simulink subsystem "thermal_controller_standalone"  (R2022b)
settings: Solver=VariableStepAuto  StartTime=0.0  StopTime=10.0  RelTol=1e-3
libraries: slpidlib x1
settings Model: Creator=michael.roesch  LastModifiedBy=stefan.notter

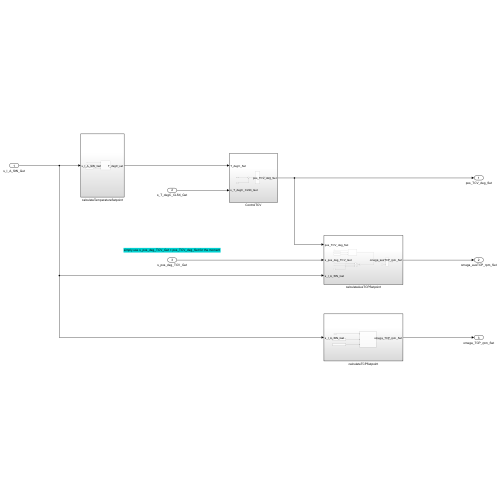
[thumbnail: Simulink's stored preview of the top-level diagram]
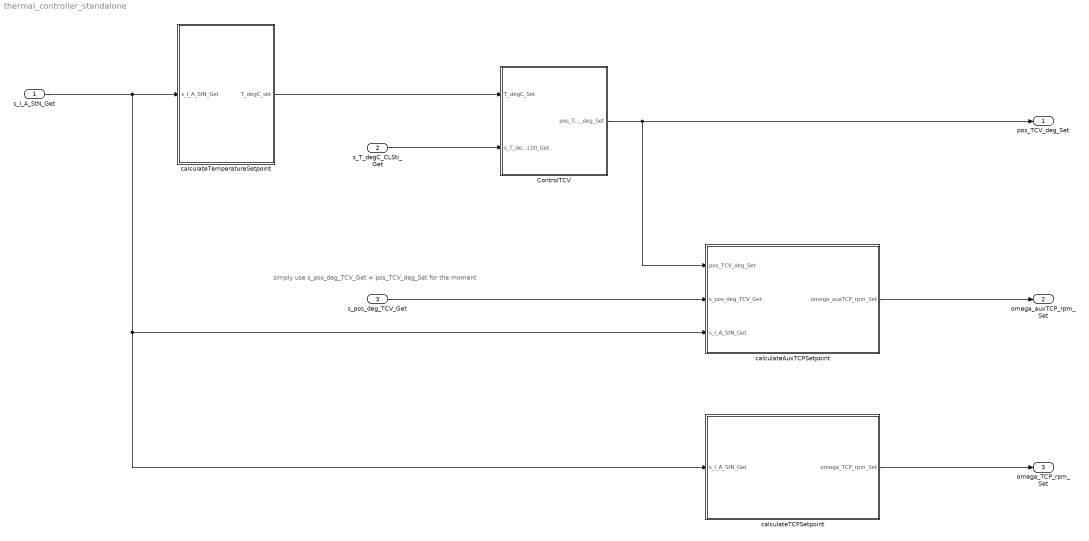
== system thermal_controller_standalone ==
  note: simply use s_pos_deg_TCV_Get = pos_TCV_deg_Set for the moment
  s_I_A_StN_Get : Inport
  s_T_degC_CLSti_Get : Inport  Port=2
  s_pos_deg_TCV_Get : Inport  Port=3
  ControlTCV : Subsystem
  calculateAuxTCPSetpoint : Subsystem
  calculateTCPSetpoint : Subsystem
  calculateTemperatureSetpoint : Subsystem
  pos_TCV_deg_Set : Outport
  omega_auxTCP_rpm_Set : Outport  Port=2
  omega_TCP_rpm_Set : Outport  Port=3
  wires:
  calculateTemperatureSetpoint/1(T_degC_set) -> ControlTCV/1(T_degC_Set)
  calculateTCPSetpoint/1(omega_TCP_rpm_Set) -> omega_TCP_rpm_Set/1
  calculateAuxTCPSetpoint/1(omega_auxTCP_rpm_Set) -> omega_auxTCP_rpm_Set/1
  ControlTCV/1(pos_TCV_deg_Set) -> pos_TCV_deg_Set/1, calculateAuxTCPSetpoint/1(pos_TCV_deg_Set)
  s_I_A_StN_Get/1 -> calculateTCPSetpoint/1(s_I_A_StN_Get), calculateAuxTCPSetpoint/3(s_I_A_StN_Get), calculateTemperatureSetpoint/1(s_I_A_StN_Get)
  s_T_degC_CLSti_Get/1 -> ControlTCV/2(s_T_degC_CLSti_Get)
  s_pos_deg_TCV_Get/1 -> calculateAuxTCPSetpoint/2(s_pos_deg_TCV_Get)

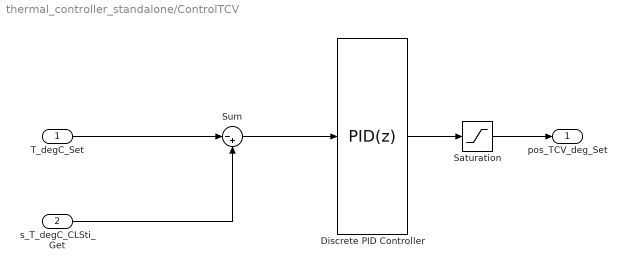
== system thermal_controller_standalone/ControlTCV ==
  T_degC_Set : Inport
  s_T_degC_CLSti_Get : Inport  Port=2
  Discrete PID Controller : slpidlib/PID Controller  Controller=PID  Form=Parallel  TimeDomain=Discrete-time  UseExternalTs=off  SampleTime=-1  IntegratorMethod=Forward Euler  FilterMethod=Forward Euler  ControllerParametersSource=internal  P=500  I=1  UseKiTs=on  D=0  N=0  UseFilter=on  TunerSelectOption=Transfer Function Based (PID Tuner App)  InitialConditionSource=internal  InitialConditionForIntegrator=0  InitialConditionForFilter=0  DifferentiatorICPrevScaledInput=0  ExternalReset=none  TrackingMode=off  Kt=1  LimitOutput=off  SatLimitsSource=internal  UpperSaturationLimit=90  LowerSaturationLimit=25  LinearizeAsGain=on  AntiWindupMode=clamping  Kb=1  LimitIntegrator=off  UpperIntegratorSaturationLimit=inf  LowerIntegratorSaturationLimit=-inf  POutMin=[]  POutMax=[]  IOutMin=[]  IOutMax=[]  DOutMin=[]  DOutMax=[]  NOutMin=[]  NOutMax=[]  SumOutMin=[]  SumOutMax=[]  SaturationOutMin=[]  SaturationOutMax=[]  PParamMin=[]  PParamMax=[]  IParamMin=[]  IParamMax=[]  DParamMin=[]  DParamMax=[]  NParamMin=[]  NParamMax=[]  KbParamMin=[]  KbParamMax=[]  KtParamMin=[]  KtParamMax=[]  KbOutMin=[]  KbOutMax=[]  KtOutMin=[]  KtOutMax=[]  IntegratorOutMin=[]  IntegratorOutMax=[]  FilterOutMin=[]  FilterOutMax=[]  SumI1OutMin=[]  SumI1OutMax=[]  SumI2OutMin=[]  SumI2OutMax=[]  SumI3OutMin=[]  SumI3OutMax=[]  SumI4OutMin=[]  SumI4OutMax=[]  SumDOutMin=[]  SumDOutMax=[]  DifferentiatorOutMin=[]  DifferentiatorOutMax=[]  FilterDiffOutCoefMin=[]  FilterDiffOutCoefMax=[]  ReciprocalOutMin=[]  ReciprocalOutMax=[]  SumDenOutMin=[]  SumDenOutMax=[]  SumNumOutMin=[]  SumNumOutMax=[]  DivideOutMin=[]  DivideOutMax=[]  UdiffTsProdOutMin=[]  UdiffTsProdOutMax=[]  NTsProdOutMin=[]  NTsProdOutMax=[]  UintegralTsProdOutMin=[]  UintegralTsProdOutMax=[]  UngainTsProdOutMin=[]  UngainTsProdOutMax=[]  ClampingZeroOutDataTypeStr=Inherit: Inherit via back propagation  ClampingZeroOutMin=[]  ClampingZeroOutMax=[]  FilterDenConstantOutDataTypeStr=Inherit: Inherit via back propagation  FilterDenConstantOutMin=[]  FilterDenConstantOutMax=[]  PCopyOutDataTypeStr=Inherit: Inherit via back propagation  PCopyOutMin=[]  PCopyOutMax=[]  NCopyOutDataTypeStr=Inherit: Inherit via back propagation  NCopyOutMin=[]  NCopyOutMax=[]  IntegratorContinuousStateAttributes=''  IntegratorStateMustResolveToSignalObject=off  IntegratorRTWStateStorageClass=Auto  FilterContinuousStateAttributes=''  FilterStateMustResolveToSignalObject=off  FilterRTWStateStorageClass=Auto  ParallelPVariant=InternalParameters  IdealPVariant=Disabled  IVariant=InternalParameters  DVariant=InternalParameters  IntegratorVariant=Discrete  SatVariant=Disabled  AWVariant=Passthrough  PCopyVariant=Disabled  TRVariant=Disabled  FdbkBlocksVariant=Forward  IdealPFdbkVariant=Disabled  SatFdbkVariant=Disabled  DerivativeFilterVariant=ForwardEulerFilter  NVariant=InternalParameters  NCopyVariant=Disabled  FilterICVariant=InternalICsFilter  IntegratorICVariant=InternalICs  ExternalResetVariant=Disabled  TRSumVariant=Passthrough  SumFdbkVariant=Disabled  SumVariant=Sum_PID  TsampFilterVariant=InternalTs  TsampNgainVariant=Passthrough  TsampIntegralVariant=Passthrough  ExternalSaturationOutDataTypeStr=Inherit: Same as second input
      settings: LibrarySourceBlock=simulink/Discrete/Discrete PID Controller
  Saturation : Saturate  UpperLimit=90  LowerLimit=25
  Sum : Sum  Inputs=|-+
  pos_TCV_deg_Set : Outport
  wires:
  T_degC_Set/1 -> Sum/1
  Discrete PID Controller/1 -> Saturation/1
  Sum/1 -> Discrete PID Controller/1
  s_T_degC_CLSti_Get/1 -> Sum/2
  Saturation/1 -> pos_TCV_deg_Set/1

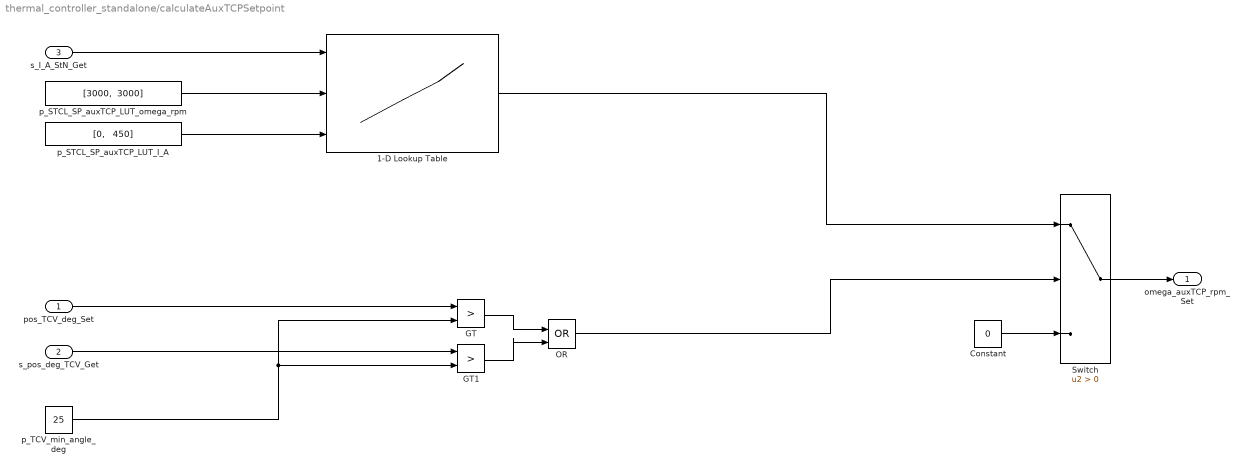
== system thermal_controller_standalone/calculateAuxTCPSetpoint ==
  pos_TCV_deg_Set : Inport
  s_pos_deg_TCV_Get : Inport  Port=2
  s_I_A_StN_Get : Inport  Port=3
  1-D Lookup Table : Lookup_n-D  NumberOfTableDimensions=1  BreakpointsForDimension1Source=Input port  BreakpointsForDimension1=[-5:5]  TableSource=Input port  Table=tanh([-5:5])  InternalRulePriority=Speed  RndMeth=Simplest
      settings: InputPortMap=u0,p221,p5
  Constant : Constant  Value=0
  GT : RelationalOperator  Operator=>  OutDataTypeStr=boolean  RndMeth=Simplest  InputSameDT=off
  GT1 : RelationalOperator  Operator=>  OutDataTypeStr=boolean  RndMeth=Simplest  InputSameDT=off
  OR : Logic  Operator=OR  IconShape=distinctive  AllPortsSameDT=off  OutDataTypeStr=boolean
  Switch : Switch  Criteria=u2 > Threshold  SaturateOnIntegerOverflow=off  InputSameDT=off
  p_STCL_SP_auxTCP_LUT_I_A : Constant  Value="[0,   450]"
  p_STCL_SP_auxTCP_LUT_omega_rpm : Constant  Value="[3000,  3000]"
  p_TCV_min_angle_deg : Constant  Value=25
  omega_auxTCP_rpm_Set : Outport
  wires:
  Constant/1 -> Switch/3
  OR/1 -> Switch/2
  GT1/1 -> OR/2
  GT/1 -> OR/1
  pos_TCV_deg_Set/1 -> GT/1
  s_I_A_StN_Get/1 -> 1-D Lookup Table/1
  Switch/1 -> omega_auxTCP_rpm_Set/1
  1-D Lookup Table/1 -> Switch/1
  p_STCL_SP_auxTCP_LUT_omega_rpm/1 -> 1-D Lookup Table/2
  p_STCL_SP_auxTCP_LUT_I_A/1 -> 1-D Lookup Table/3
  s_pos_deg_TCV_Get/1 -> GT1/1
  p_TCV_min_angle_deg/1 -> GT/2, GT1/2

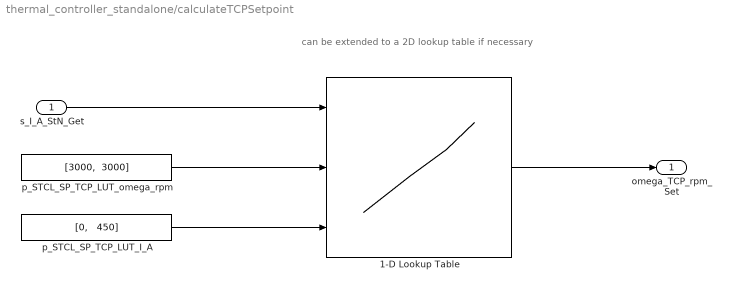
== system thermal_controller_standalone/calculateTCPSetpoint ==
  note: can be extended to a 2D lookup table if necessary
  s_I_A_StN_Get : Inport
  1-D Lookup Table : Lookup_n-D  NumberOfTableDimensions=1  BreakpointsForDimension1Source=Input port  BreakpointsForDimension1=[-5:5]  TableSource=Input port  Table=tanh([-5:5])  InternalRulePriority=Speed  RndMeth=Simplest
      settings: InputPortMap=u0,p221,p5
  p_STCL_SP_TCP_LUT_I_A : Constant  Value="[0,   450]"
  p_STCL_SP_TCP_LUT_omega_rpm : Constant  Value="[3000,  3000]"
  omega_TCP_rpm_Set : Outport
  wires:
  1-D Lookup Table/1 -> omega_TCP_rpm_Set/1
  s_I_A_StN_Get/1 -> 1-D Lookup Table/1
  p_STCL_SP_TCP_LUT_omega_rpm/1 -> 1-D Lookup Table/2
  p_STCL_SP_TCP_LUT_I_A/1 -> 1-D Lookup Table/3

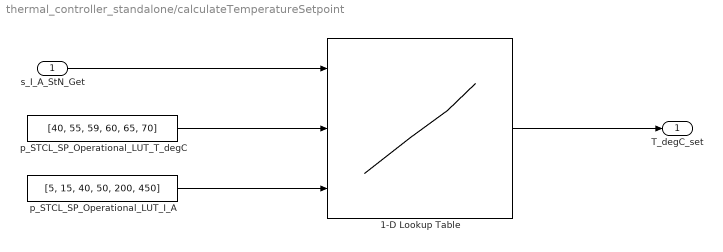
== system thermal_controller_standalone/calculateTemperatureSetpoint ==
  s_I_A_StN_Get : Inport
  1-D Lookup Table : Lookup_n-D  NumberOfTableDimensions=1  BreakpointsForDimension1Source=Input port  BreakpointsForDimension1=[-5:5]  TableSource=Input port  Table=tanh([-5:5])  InternalRulePriority=Speed  RndMeth=Simplest
      settings: InputPortMap=u0,p221,p5
  p_STCL_SP_Operational_LUT_I_A : Constant  Value="[5,   15,     40,     50,     200,    450]"
  p_STCL_SP_Operational_LUT_T_degC : Constant  Value="[40,  55,\t    59,     60,     65,\t    70]"
  T_degC_set : Outport
  wires:
  s_I_A_StN_Get/1 -> 1-D Lookup Table/1
  1-D Lookup Table/1 -> T_degC_set/1
  p_STCL_SP_Operational_LUT_T_degC/1 -> 1-D Lookup Table/2
  p_STCL_SP_Operational_LUT_I_A/1 -> 1-D Lookup Table/3
